simulink model "animation11"  (R2021b)
settings: Solver=ode3  StartTime=0  StopTime=10  FixedStep=0.001  RelTol=1e-3
settings Model: Creator=hukai  LastModifiedBy=hukai

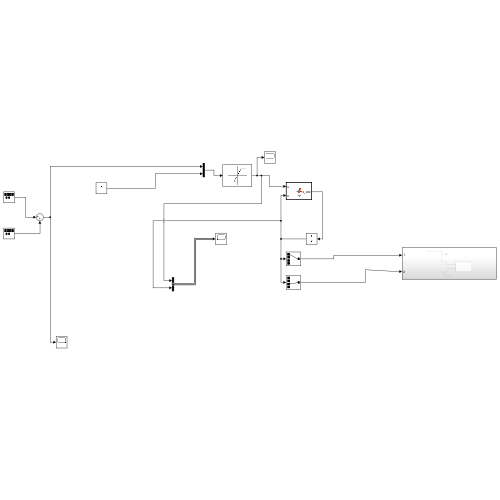
[thumbnail: Simulink's stored preview of the top-level diagram]
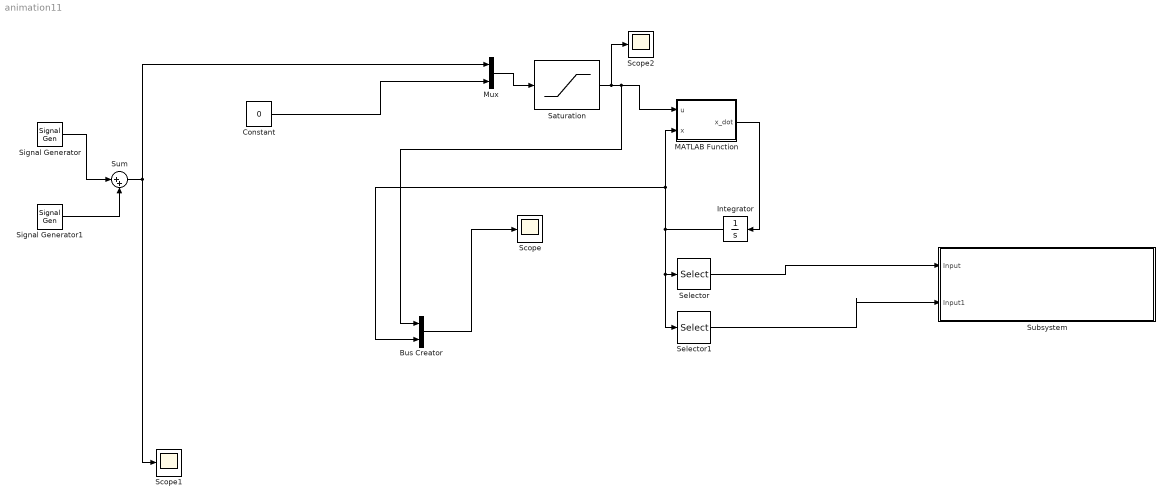
== system animation11 ==
  Bus Creator : BusCreator  Inputs=2
  Constant : Constant  Value=0
  Integrator : Integrator  InitialCondition=[0;0;-180;0]
  MATLAB Function : MATLAB Function  TreatAsAtomicUnit=on
  Mux : Mux  Inputs=2
  Saturation : Saturate
  Scope : Scope
  Scope1 : Scope
  Scope2 : Scope
  Selector : Selector  InputPortWidth=4  IndexOptions=Index vector (dialog)  Indices=[1]  OutputSizes=1
  Selector1 : Selector  InputPortWidth=4  IndexOptions=Index vector (dialog)  Indices=[3]  OutputSizes=1
  Signal Generator : SignalGenerator  Amplitude=2*pi  Frequency=0.1  Units=rad/sec
  Signal Generator1 : SignalGenerator  WaveForm=square  Amplitude=100  Frequency=2.5  Units=rad/sec
  Subsystem : Subsystem
  Sum : Sum  Inputs=|++
  wires:
  MATLAB Function/1(x_dot) -> Integrator/1
  Integrator/1 -> Bus Creator/2, MATLAB Function/2(x), Selector1/1, Selector/1
  Selector1/1 -> Subsystem/2(Input1)
  Selector/1 -> Subsystem/1(Input)
  Constant/1 -> Mux/2
  Bus Creator/1 -> Scope/1
  Sum/1 -> Scope1/1, Mux/1
  Mux/1 -> Saturation/1
  Saturation/1 -> Scope2/1, Bus Creator/1, MATLAB Function/1(u)
  Signal Generator/1 -> Sum/1
  Signal Generator1/1 -> Sum/2

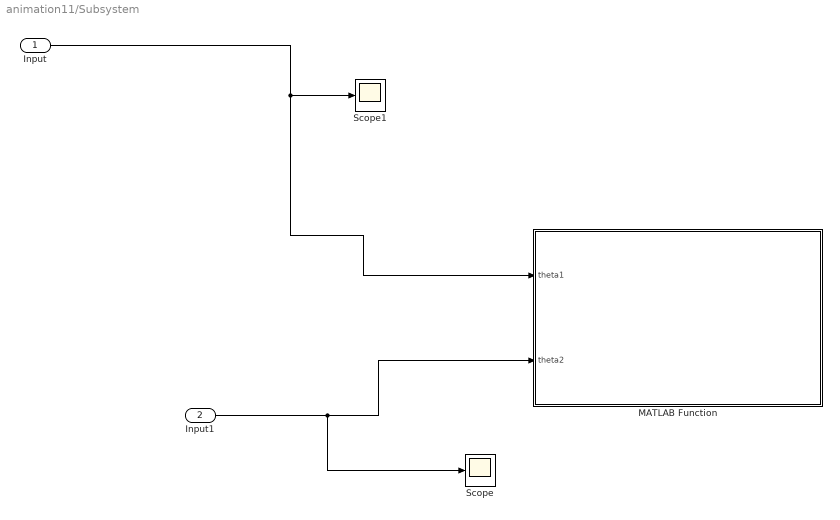
== system animation11/Subsystem ==
  Input : Inport
  Input1 : Inport  Port=2
  MATLAB Function : MATLAB Function  TreatAsAtomicUnit=on
  Scope : Scope
  Scope1 : Scope
  wires:
  Input/1 -> MATLAB Function/1(theta1), Scope1/1
  Input1/1 -> Scope/1, MATLAB Function/2(theta2)

== matlab function animation11/Subsystem/MATLAB Function ==
  data: theta1 input; theta2 input
function  fcn(theta1,theta2)
link1_frame1 = [0,0,0;
                0,0,-1;
                0,6,-1;
                0,6,0;
                0,8,0]; % declaration of link1 points in FRAME-1
link1_frame0 = zeros(5,3);
link2_frame2 = [0,0,0;
                0,12,0]; % declaration of link2 points in FRAME-1    
link2_frame1 = zeros(2,3);
link2_frame0 = zeros(2,3);
%plot3([0,0],[0,0],[-10,0],'ks-','LineWidth',1) % drawing of robot base in FRAME-0
%hold on
for i = 1:length(link1_frame1(:,1))
    link1_frame0(i,:) = TRANS0_1(link1_frame1(i,:),theta1); 
    % transformation of link1 points from FRAME-1 to FRAME-0
end
%plot3(link1_frame0(:,1),link1_frame0(:,2),link1_frame0(:,3),'bs-','LineWidth',1)
for i = 1:length(link2_frame2(:,1))
    link2_frame1(i,:) = TRANS1_2(link2_frame2(i,:),theta2,6,2);
    link2_frame0(i,:) = TRANS0_1(link2_frame1(i,:),theta1);
end
% plot3(link2_frame0(:,1),link2_frame0(:,2),link2_frame0(:,3),'rs-','LineWidth',1)
% hold off
% grid on
% axis([-15 15 -15 15 -15 15])
% title('Drawing of Base and Links 1-2 in FRAME-0 animating') 
% pause(0.001)

function fr0 = TRANS0_1(fr1, theta1)
fr1_cat = cat(2,fr1,1)';
% creates a usable 4-vector by concatination and transpose
T0_1 = [cos(theta1),-sin(theta1),0,0;
        sin(theta1),cos(theta1),0,0;
        0,0,1,0;
        0,0,0,1];
fr0_cat = (T0_1*fr1_cat);
fr0 = fr0_cat(1:3)';
end

function fr1 = TRANS1_2(fr2, theta2, l1, l2)
fr2_cat = cat(2,fr2,1)';
% creates a usable 4-vector by concatination and transpose
T1_2 = [cos(theta2),-sin(theta2),0,0;
        0,0,-1,l1+l2;
        sin(theta2),cos(theta2),0,0;
        0,0,0,1];
fr1_cat = (T1_2*fr2_cat);
fr1 = fr1_cat(1:3)';
end
% drawing link2 points and segments in FRAME-0

end

== matlab function animation11/MATLAB Function ==
  data: u input; x_dot output; x input
function x_dot  = fcn(u, x)

theta_1_dot = 0.0171;
theta_2_dot = 0.0038;
theta_3_dot = 0.0038;
theta_4_dot = 0.0921;

theta_1 = 0.0304;
theta_2 = 0.0184;
theta_3 = 0.0184;
theta_4 = 0.0921;
theta_5 = 0.6101;
theta_6 = 0.0097;

q_1 = x(1);
q_1_dot = x(2);
q_2= x(3);
q_2_dot=x(4);
q_dot = [q_1_dot;q_2_dot];

m_11 = theta_1+theta_2*sin(q_2)^2;
m_12 = theta_3*cos(q_2);
c_11 = 2*theta_2*sin(q_2)*cos(q_2)*q_2_dot;
c_12 = -theta_3*sin(q_2)*q_2_dot;
f_1 = theta_5*q_1_dot;
g_1 = 0;

m_21 = theta_3*cos(q_2);
m_22 = theta_2;
c_21 = -theta_2*sin(q_2)*cos(q_2)*q_1_dot;
c_22 = 0;
f_2 = theta_6*q_2_dot;
g_2 = 9.8*-theta_4*sin(q_2);

M = [m_11,m_12;m_21,m_22];
C = [c_11,c_12;c_21,c_22];
F = [f_1;f_2];
G = [g_1;g_2];
q_ddot = M^(-1)*(u-C*q_dot-F-G);
q_1_ddot = q_ddot(1);
q_2_ddot = q_ddot(2);
x_dot = [q_1_dot;
         q_1_ddot;
         q_2_dot;
         q_2_ddot;];
